simulink model "induction_machine_qd0"  (R2021b)
settings: Solver=FixedStepDiscrete  StartTime=0.0  StopTime=0.5  FixedStep=Ts  RelTol=1e-3
InitFcn:
  | Ts=1e-5;
  | Fe=50;
  | Vrms=230;
undefined symbols (not defined in the file): DiscIntNeverNeededParam
settings Model: Creator=lecci  LastModifiedBy=lecci

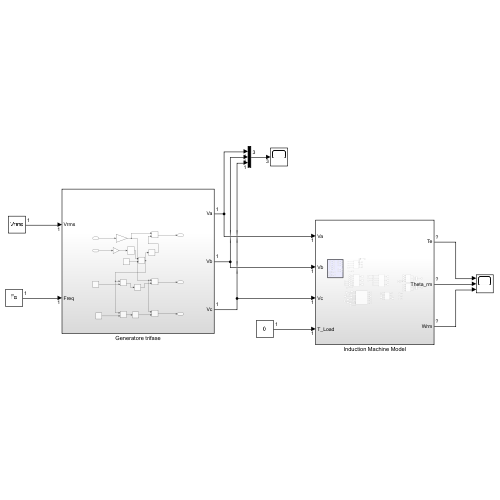
[thumbnail: Simulink's stored preview of the top-level diagram]
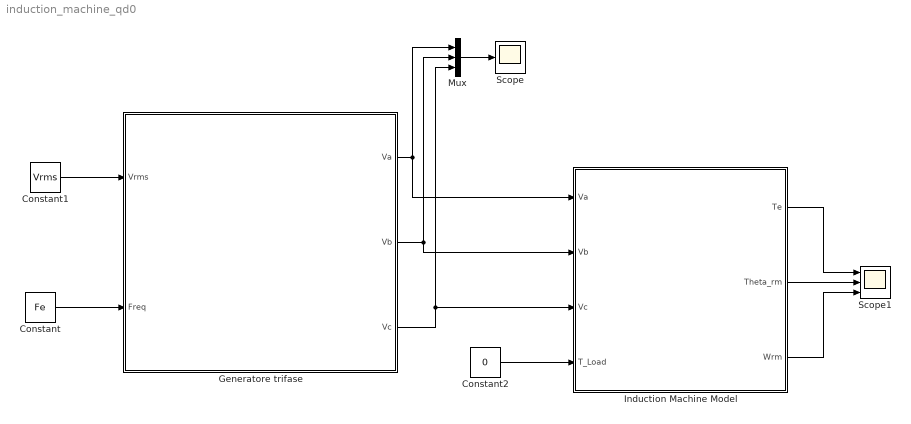
== system induction_machine_qd0 ==
  Constant : Constant  Value=Fe
  Constant1 : Constant  Value=Vrms
  Constant2 : Constant  Value=0
  Generatore trifase : Subsystem
  Induction Machine Model : Subsystem
  Mux : Mux  Inputs=3
  Scope : Scope
  Scope1 : Scope  NumInputPorts=3
  wires:
  Constant/1 -> Generatore trifase/2(Freq)
  Constant1/1 -> Generatore trifase/1(Vrms)
  Generatore trifase/1(Va) -> Induction Machine Model/1(Va), Mux/1
  Generatore trifase/2(Vb) -> Induction Machine Model/2(Vb), Mux/2
  Generatore trifase/3(Vc) -> Induction Machine Model/3(Vc), Mux/3
  Mux/1 -> Scope/1
  Constant2/1 -> Induction Machine Model/4(T_Load)
  Induction Machine Model/2(Theta_rm) -> Scope1/2
  Induction Machine Model/1(Te) -> Scope1/1
  Induction Machine Model/3(Wrm) -> Scope1/3

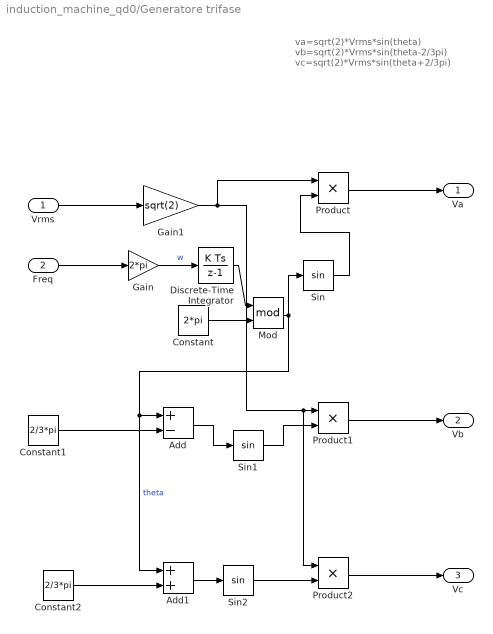
== system induction_machine_qd0/Generatore trifase ==
  note: va=sqrt(2)*Vrms*sin(theta)
      | vb=sqrt(2)*Vrms*sin(theta-2/3pi)
      | vc=sqrt(2)*Vrms*sin(theta+2/3pi)
  Vrms : Inport
  Freq : Inport  Port=2
  Add : Sum  Inputs=+-
  Add1 : Sum
  Constant : Constant  Value=2*pi
  Constant1 : Constant  Value=2/3*pi
  Constant2 : Constant  Value=2/3*pi
  Discrete-Time Integrator : DiscreteIntegrator  SampleTime=-1  ICPrevOutput=DiscIntNeverNeededParam  ICPrevScaledInput=DiscIntNeverNeededParam
  Gain : Gain  Gain=2*pi
  Gain1 : Gain  Gain=sqrt(2)
  Mod : Math  Operator=mod  SaturateOnIntegerOverflow=on
  Product : Product
  Product1 : Product
  Product2 : Product
  Sin : Trigonometry
  Sin1 : Trigonometry
  Sin2 : Trigonometry
  Va : Outport
  Vb : Outport  Port=2
  Vc : Outport  Port=3
  wires:
  Freq/1 -> Gain/1
  Constant/1 -> Mod/2
  Gain/1 -> Discrete-Time Integrator/1  "w"
  Discrete-Time Integrator/1 -> Mod/1
  Mod/1 -> Add1/1, Add/1, Sin/1  "theta"
  Sin/1 -> Product/2
  Product/1 -> Va/1
  Constant1/1 -> Add/2
  Product1/1 -> Vb/1
  Product2/1 -> Vc/1
  Constant2/1 -> Add1/2
  Gain1/1 -> Product2/1, Product1/1, Product/1
  Vrms/1 -> Gain1/1
  Add/1 -> Sin1/1
  Sin1/1 -> Product1/2
  Add1/1 -> Sin2/1
  Sin2/1 -> Product2/2

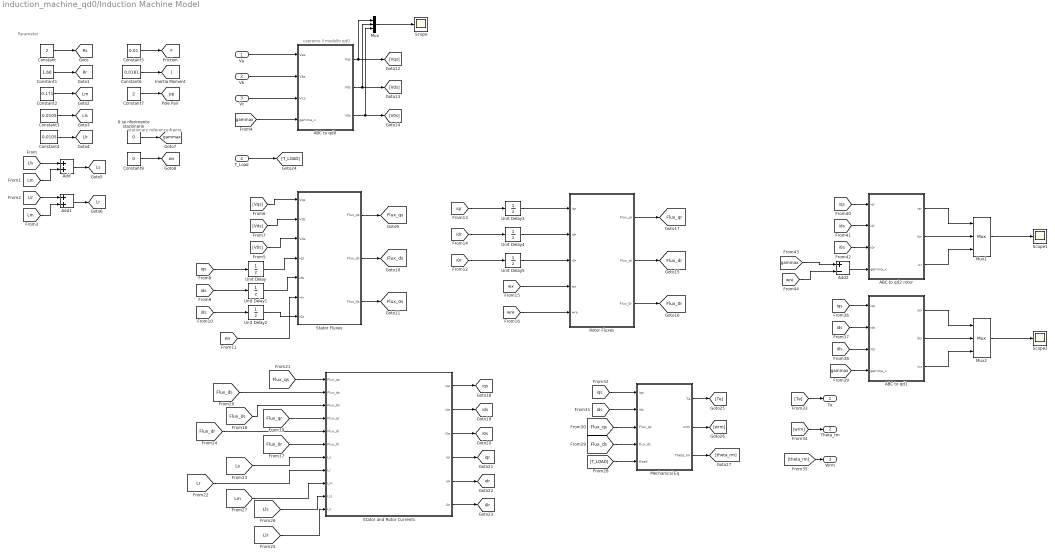
== system induction_machine_qd0/Induction Machine Model ==
  note: stationary reference frame
  note: useremo il modello qd0
  note: Parameter
  Va : Inport
  Vb : Inport  Port=2
  Vc : Inport  Port=3
  T_Load : Inport  Port=4
  0 se riferimento stazionario : Constant  Value=0
  ABC to qd0 : MATLAB Function  TreatAsAtomicUnit=on
  ABC to qd1 : MATLAB Function  TreatAsAtomicUnit=on
  ABC to qd2 rotor : MATLAB Function  TreatAsAtomicUnit=on
  Add : Sum
  Add1 : Sum
  Add2 : Sum  Inputs=+-
  Constant : Constant  Value=2
  Constant1 : Constant  Value=1.66
  Constant2 : Constant  Value=0.171
  Constant3 : Constant  Value=0.0105
  Constant4 : Constant  Value=0.0105
  Constant5 : Constant  Value=0.01
  Constant6 : Constant  Value=0.0181
  Constant7 : Constant  Value=2
  Constant9 : Constant  Value=0
  Mechanical Eq : Subsystem
  Mux : Mux  Inputs=3
  Mux1 : Mux  Inputs=3
  Mux2 : Mux  Inputs=3
  Rotor Fluxes : Subsystem
  Scope : Scope
  Scope1 : Scope
  Scope2 : Scope
  Stator Fluxes : Subsystem
  Stator and Rotor Currents : MATLAB Function  TreatAsAtomicUnit=on
  Unit Delay{,1..5} (6 alike) : UnitDelay  SampleTime=-1  HasFrameUpgradeWarning=on
  Te : Outport
  Theta_rm : Outport  Port=2
  Wrm : Outport  Port=3
  tag scope: F=global, Flux_0r=global, Flux_0s=global, Flux_dr=global, Flux_ds=global, Flux_qr=global, Flux_qs=global, J=global, Llr=global, Lls=global, Lm=global, Lr=global, Ls=global, Rr=global, Rs=global, gammax=global, i0r=global, i0s=global, idr=global, ids=global, iqr=global, iqs=global, pp=global, wx=global
  wires:
  Constant/1 -> [Rs]
  Constant1/1 -> [Rr]
  Constant2/1 -> [Lm]
  Constant3/1 -> [Lls]
  Constant4/1 -> [Llr]
  Add/1 -> [Ls]
  [Lls] -> Add/1
  [Lm] -> Add/2
  Add1/1 -> [Lr]
  [Llr] -> Add1/1
  [Lm] -> Add1/2
  Constant5/1 -> [F]
  Constant6/1 -> [J]
  Constant7/1 -> [pp]
  Va/1 -> ABC to qd0/1(Vas)
  Vb/1 -> ABC to qd0/2(Vbs)
  Vc/1 -> ABC to qd0/3(Vcs)
  0 se riferimento stazionario/1 -> [gammax]
  [gammax] -> ABC to qd0/4(gamma_x)
  Constant9/1 -> [wx]
  ABC to qd0/1(Vqs) -> [Vqs], Mux/1
  ABC to qd0/2(Vds) -> [Vds], Mux/2
  ABC to qd0/3(V0s) -> [V0s], Mux/3
  Mux/1 -> Scope/1
  Stator Fluxes/1(Flux_qs) -> [Flux_qs]
  Stator Fluxes/2(Flux_ds) -> [Flux_ds]
  Stator Fluxes/3(Flux_0s) -> [Flux_0s]
  [V0s] -> Stator Fluxes/3(V0s)
  [Vqs] -> Stator Fluxes/1(Vqs)
  [Vds] -> Stator Fluxes/2(Vds)
  [i0s] -> Unit Delay2/1
  Unit Delay2/1 -> Stator Fluxes/7(i0s)
  [ids] -> Unit Delay1/1
  [iqs] -> Unit Delay/1
  Unit Delay/1 -> Stator Fluxes/4(iqs)
  Unit Delay1/1 -> Stator Fluxes/5(ids)
  [wx] -> Stator Fluxes/6(wx)
  [idr] -> Unit Delay4/1
  [i0r] -> Unit Delay5/1
  [iqr] -> Unit Delay3/1
  Unit Delay3/1 -> Rotor Fluxes/1(iqr)
  Unit Delay4/1 -> Rotor Fluxes/2(idr)
  Unit Delay5/1 -> Rotor Fluxes/3(i0r)
  [wx] -> Rotor Fluxes/4(wx)
  [wre] -> Rotor Fluxes/5(wre)
  Rotor Fluxes/1(Flux_qr) -> [Flux_qr]
  Rotor Fluxes/2(Flux_dr) -> [Flux_dr]
  Rotor Fluxes/3(Flux_0r) -> [Flux_0r]
  Stator and Rotor Currents/1(iqs) -> [iqs]
  Stator and Rotor Currents/3(i0s) -> [i0s]
  Stator and Rotor Currents/2(ids) -> [ids]
  Stator and Rotor Currents/4(iqr) -> [iqr]
  Stator and Rotor Currents/5(idr) -> [idr]
  Stator and Rotor Currents/6(i0r) -> [i0r]
  [Flux_0r] -> Stator and Rotor Currents/6(Flux_0r)
  [Flux_ds] -> Stator and Rotor Currents/2(Flux_ds)
  [Flux_qs] -> Stator and Rotor Currents/1(Flux_qs)
  [Flux_0s] -> Stator and Rotor Currents/3(Flux_0s)
  [Flux_qr] -> Stator and Rotor Currents/4(Flux_qr)
  [Flux_dr] -> Stator and Rotor Currents/5(Flux_dr)
  [Ls] -> Stator and Rotor Currents/7(Ls)
  [Lr] -> Stator and Rotor Currents/8(Lr)
  [Lm] -> Stator and Rotor Currents/9(Lm)
  [Lls] -> Stator and Rotor Currents/10(Lls)
  [Llr] -> Stator and Rotor Currents/11(Llr)
  T_Load/1 -> [T_LOAD]
  [T_LOAD] -> Mechanical Eq/5(tload)
  [Flux_ds] -> Mechanical Eq/4(flux_ds)
  [Flux_qs] -> Mechanical Eq/3(Flux_qs)
  [ids] -> Mechanical Eq/2(ids)
  [iqs] -> Mechanical Eq/1(iqs)
  Mechanical Eq/1(Te) -> [Te]
  Mechanical Eq/2(wrm) -> [wrm]
  Mechanical Eq/3(Theta_rm) -> [theta_rm]
  [Te] -> Te/1
  [wrm] -> Theta_rm/1
  [theta_rm] -> Wrm/1
  [iqs] -> ABC to qd1/1(iqs)
  [ids] -> ABC to qd1/2(ids)
  [i0s] -> ABC to qd1/3(i0s)
  [gammax] -> ABC to qd1/4(gamma_x)
  [iqs] -> ABC to qd2 rotor/1(iqr)
  [ids] -> ABC to qd2 rotor/2(idr)
  [i0s] -> ABC to qd2 rotor/3(i0r)
  ABC to qd2 rotor/1(iar) -> Mux1/1
  ABC to qd2 rotor/2(ibr) -> Mux1/2
  ABC to qd2 rotor/3(icr) -> Mux1/3
  Mux1/1 -> Scope1/1
  ABC to qd1/3(ics) -> Mux2/3
  Mux2/1 -> Scope2/1
  ABC to qd1/2(ibs) -> Mux2/2
  ABC to qd1/1(ias) -> Mux2/1
  Add2/1 -> ABC to qd2 rotor/4(gamma_x)
  [gammax] -> Add2/1
  [wre] -> Add2/2

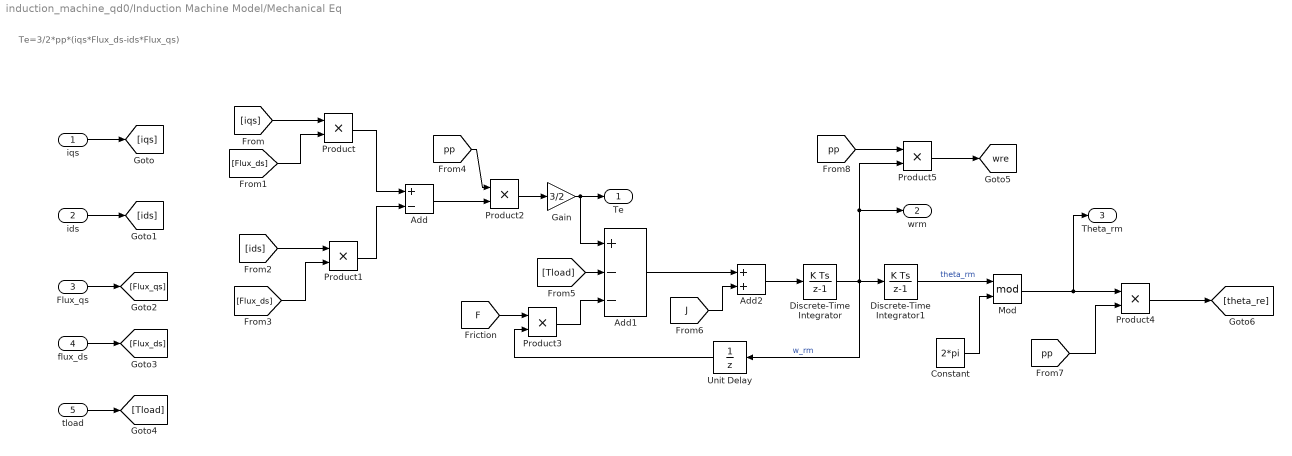
== system induction_machine_qd0/Induction Machine Model/Mechanical Eq ==
  note: Te=3/2*pp*(iqs*Flux_ds-ids*Flux_qs)
  iqs : Inport
  ids : Inport  Port=2
  Flux_qs : Inport  Port=3
  flux_ds : Inport  Port=4
  tload : Inport  Port=5
  Add : Sum  Inputs=+-
  Add1 : Sum  Inputs=+--
  Add2 : Sum
  Constant : Constant  Value=2*pi
  Discrete-Time Integrator : DiscreteIntegrator  SampleTime=-1  ICPrevOutput=DiscIntNeverNeededParam  ICPrevScaledInput=DiscIntNeverNeededParam
  Discrete-Time Integrator1 : DiscreteIntegrator  SampleTime=-1  ICPrevOutput=DiscIntNeverNeededParam  ICPrevScaledInput=DiscIntNeverNeededParam
  Gain : Gain  Gain=3/2
  Mod : Math  Operator=mod  SaturateOnIntegerOverflow=on
  Product{,1..5} (6 alike) : Product
  Unit Delay : UnitDelay  SampleTime=-1  HasFrameUpgradeWarning=on
  Te : Outport
  wrm : Outport  Port=2
  Theta_rm : Outport  Port=3
  tag scope: wre=global
  wires:
  iqs/1 -> [iqs]
  ids/1 -> [ids]
  Flux_qs/1 -> [Flux_qs]
  flux_ds/1 -> [Flux_ds]
  [iqs] -> Product/1
  [Flux_ds] -> Product/2
  Product/1 -> Add/1
  [Flux_ds] -> Product1/2
  [ids] -> Product1/1
  Product1/1 -> Add/2
  Add/1 -> Product2/2
  [pp] -> Product2/1
  Product2/1 -> Gain/1
  Gain/1 -> Add1/1, Te/1
  tload/1 -> [Tload]
  [Tload] -> Add1/2
  Product3/1 -> Add1/3
  [F] -> Product3/1
  Add1/1 -> Add2/1
  [J] -> Add2/2
  Add2/1 -> Discrete-Time Integrator/1
  Discrete-Time Integrator/1 -> Product5/2, wrm/1, Discrete-Time Integrator1/1, Unit Delay/1  "w_rm"
  Unit Delay/1 -> Product3/2
  Constant/1 -> Mod/2
  Mod/1 -> Theta_rm/1, Product4/1
  [pp] -> Product4/2
  Discrete-Time Integrator1/1 -> Mod/1  "theta_rm"
  [pp] -> Product5/1
  Product5/1 -> [wre]
  Product4/1 -> [theta_re]

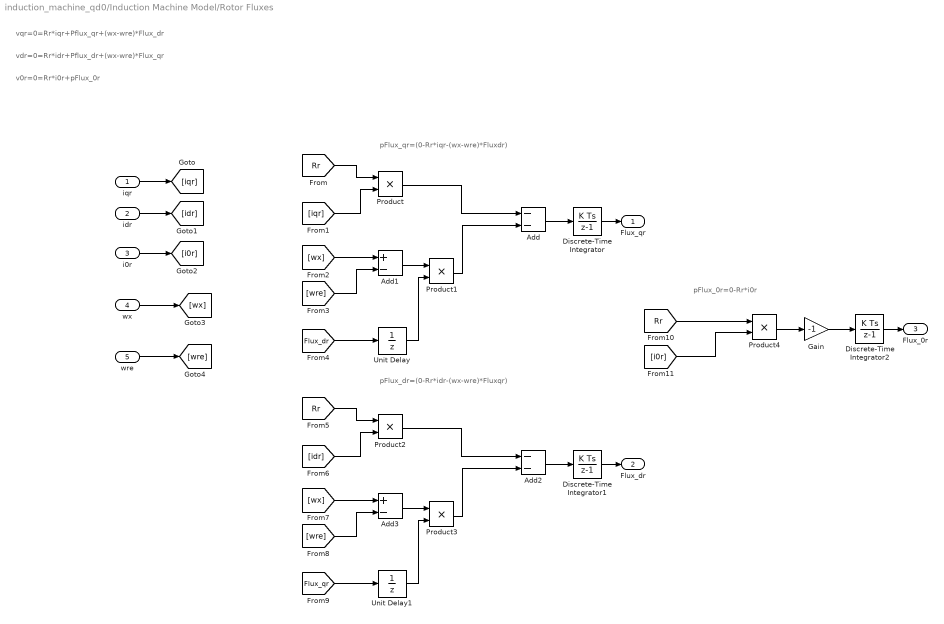
== system induction_machine_qd0/Induction Machine Model/Rotor Fluxes ==
  note: pFlux_0r=0-Rr*i0r
  note: pFlux_dr=(0-Rr*idr-(wx-wre)*Fluxqr)
  note: pFlux_qr=(0-Rr*iqr-(wx-wre)*Fluxdr)
  note: v0r=0=Rr*i0r+pFlux_0r
  note: vdr=0=Rr*idr+Pflux_dr+(wx-wre)*Flux_qr
  note: vqr=0=Rr*iqr+Pflux_qr+(wx-wre)*Flux_dr
  iqr : Inport
  idr : Inport  Port=2
  i0r : Inport  Port=3
  wx : Inport  Port=4
  wre : Inport  Port=5
  Add : Sum  Inputs=--
  Add1 : Sum  Inputs=+-
  Add2 : Sum  Inputs=--
  Add3 : Sum  Inputs=+-
  Discrete-Time Integrator : DiscreteIntegrator  SampleTime=-1  ICPrevOutput=DiscIntNeverNeededParam  ICPrevScaledInput=DiscIntNeverNeededParam
  Discrete-Time Integrator1 : DiscreteIntegrator  SampleTime=-1  ICPrevOutput=DiscIntNeverNeededParam  ICPrevScaledInput=DiscIntNeverNeededParam
  Discrete-Time Integrator2 : DiscreteIntegrator  SampleTime=-1  ICPrevOutput=DiscIntNeverNeededParam  ICPrevScaledInput=DiscIntNeverNeededParam
  Gain : Gain  Gain=-1
  Product{,1..4} (5 alike) : Product
  Unit Delay : UnitDelay  SampleTime=-1  HasFrameUpgradeWarning=on
  Unit Delay1 : UnitDelay  SampleTime=-1  HasFrameUpgradeWarning=on
  Flux_qr : Outport
  Flux_dr : Outport  Port=2
  Flux_0r : Outport  Port=3
  wires:
  iqr/1 -> [iqr]
  idr/1 -> [idr]
  i0r/1 -> [i0r]
  wx/1 -> [wx]
  wre/1 -> [wre]
  [Rr] -> Product/1
  [iqr] -> Product/2
  Product/1 -> Add/1
  [wx] -> Add1/1
  [wre] -> Add1/2
  Add1/1 -> Product1/1
  Product1/1 -> Add/2
  Add/1 -> Discrete-Time Integrator/1
  Discrete-Time Integrator/1 -> Flux_qr/1
  Product3/1 -> Add2/2
  Product2/1 -> Add2/1
  [wx] -> Add3/1
  Discrete-Time Integrator1/1 -> Flux_dr/1
  [wre] -> Add3/2
  [Rr] -> Product2/1
  Add2/1 -> Discrete-Time Integrator1/1
  [idr] -> Product2/2
  Add3/1 -> Product3/1
  Discrete-Time Integrator2/1 -> Flux_0r/1
  Gain/1 -> Discrete-Time Integrator2/1
  Product4/1 -> Gain/1
  [Rr] -> Product4/1
  [i0r] -> Product4/2
  Unit Delay/1 -> Product1/2
  [Flux_dr] -> Unit Delay/1
  [Flux_qr] -> Unit Delay1/1
  Unit Delay1/1 -> Product3/2

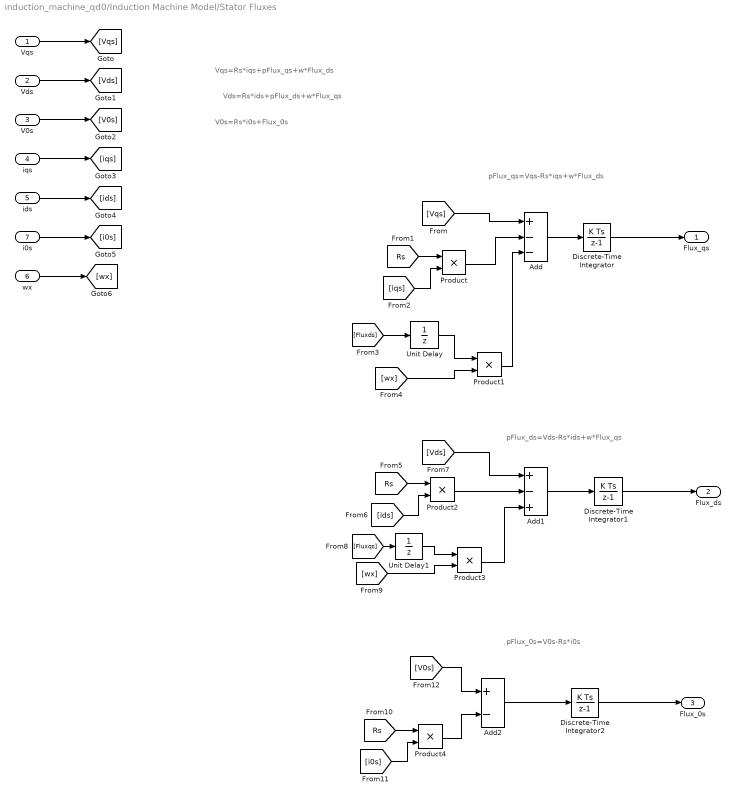
== system induction_machine_qd0/Induction Machine Model/Stator Fluxes ==
  note: pFlux_0s=V0s-Rs*i0s
  note: pFlux_qs=Vqs-Rs*iqs+w*Flux_ds
  note: pFlux_ds=Vds-Rs*ids+w*Flux_qs
  note: V0s=Rs*i0s+Flux_0s
  note: Vds=Rs*ids+pFlux_ds+w*Flux_qs
  note: Vqs=Rs*iqs+pFlux_qs+w*Flux_ds
  Vqs : Inport
  Vds : Inport  Port=2
  V0s : Inport  Port=3
  iqs : Inport  Port=4
  ids : Inport  Port=5
  wx : Inport  Port=6
  i0s : Inport  Port=7
  Add : Sum  Inputs=+--
  Add1 : Sum  Inputs=+-+
  Add2 : Sum  Inputs=+-
  Discrete-Time Integrator : DiscreteIntegrator  SampleTime=-1  ICPrevOutput=DiscIntNeverNeededParam  ICPrevScaledInput=DiscIntNeverNeededParam
  Discrete-Time Integrator1 : DiscreteIntegrator  SampleTime=-1  ICPrevOutput=DiscIntNeverNeededParam  ICPrevScaledInput=DiscIntNeverNeededParam
  Discrete-Time Integrator2 : DiscreteIntegrator  SampleTime=-1  ICPrevOutput=DiscIntNeverNeededParam  ICPrevScaledInput=DiscIntNeverNeededParam
  Product{,1..4} (5 alike) : Product
  Unit Delay : UnitDelay  SampleTime=-1  HasFrameUpgradeWarning=on
  Unit Delay1 : UnitDelay  SampleTime=-1  HasFrameUpgradeWarning=on
  Flux_qs : Outport
  Flux_ds : Outport  Port=2
  Flux_0s : Outport  Port=3
  wires:
  Vqs/1 -> [Vqs]
  V0s/1 -> [V0s]
  iqs/1 -> [iqs]
  ids/1 -> [ids]
  i0s/1 -> [i0s]
  [Vqs] -> Add/1
  [Rs] -> Product/1
  [iqs] -> Product/2
  Product/1 -> Add/2
  [wx] -> Product1/2
  [Fluxds] -> Unit Delay/1
  Unit Delay/1 -> Product1/1
  Product1/1 -> Add/3
  Add/1 -> Discrete-Time Integrator/1
  Discrete-Time Integrator/1 -> Flux_qs/1
  [Rs] -> Product2/1
  [ids] -> Product2/2
  Product2/1 -> Add1/2
  [Vds] -> Add1/1
  [Fluxqs] -> Unit Delay1/1
  [wx] -> Product3/2
  Unit Delay1/1 -> Product3/1
  Product3/1 -> Add1/3
  Discrete-Time Integrator1/1 -> Flux_ds/1
  Add1/1 -> Discrete-Time Integrator1/1
  Add2/1 -> Discrete-Time Integrator2/1
  Discrete-Time Integrator2/1 -> Flux_0s/1
  [i0s] -> Product4/2
  [Rs] -> Product4/1
  [V0s] -> Add2/1
  Product4/1 -> Add2/2
  Vds/1 -> [Vds]
  wx/1 -> [wx]

== matlab function induction_machine_qd0/Induction Machine Model/Stator and Rotor Currents ==
  data: Flux_qs input; iqs output; Flux_ds input; Flux_0s input; Flux_qr input; Flux_dr input; Flux_0r input; Ls input; Lr input; Lm input; ids output; i0s output; iqr output; idr output; i0r output; Lls input; Llr input
function [iqs,ids,i0s,iqr,idr,i0r] = fcn(Flux_qs,Flux_ds,Flux_0s,Flux_qr,Flux_dr,Flux_0r,Ls,Lr,Lm,Lls,Llr)

Flux=[Flux_qs; Flux_ds;Flux_qr;Flux_dr]

L=[Ls 0 Lm 0;
    0 Ls 0 Lm;
    Lm 0 Lr 0;
    0 Lm 0 Lr]

iqd=inv(L)*Flux;

iqs=idq(1);
ids=iqd(2);
iqr=iqd(3);
idr=iqd(4);

i0s=Flux_0s/Lls;
i0r=Flux_0r/Llr;

== matlab function induction_machine_qd0/Induction Machine Model/ABC to qd0 ==
  data: Vas input; Vqs output; Vbs input; Vcs input; gamma_x input; Vds output; V0s output
function [Vqs,Vds,V0s] = fcn(Vas,Vbs,Vcs,gamma_x)

Vabcs=[Vas;Vbs;Vcs];

K=2/3*[cos(gamma_x) cos(gamma_x-2/3*pi) cos(gamma_x+2/3*pi);
       sin(gamma_x) sin(gamma_x-2/3*pi) sin(gamma_x+2/3*pi);
       1/2                1/2                1/2     ];

Vqds=K*Vabcs;

Vqs=Vqds(1);
Vds=Vqds(2);
V0s=Vqds(3);

== matlab function induction_machine_qd0/Induction Machine Model/ABC to qd1 ==
  data: iqs input; ias output; ids input; i0s input; gamma_x input; ibs output; ics output
function [ias,ibs,ics] = fcn(iqs,ids,i0s,gamma_x)

Iqd0s=[iqs;ids;i0s];

invK=[cos(gamma_x) sin(gamma_x) 1;
       cos(gamma_x-2/3*pi) sin(gamma_x-2/3*pi) 1;
       cos(gamma_x+2/3*pi) sin(gamma_x+2/3*pi) 1];

Iabcs=invK*Iqd0s;

ias=Iabcs(1);
ibs=Iabcs(2);
ics=Iabcs(3);

== matlab function induction_machine_qd0/Induction Machine Model/ABC to qd2 rotor ==
  data: iqr input; iar output; idr input; i0r input; gamma_x input; ibr output; icr output
function [iar,ibr,icr] = fcn(iqr,idr,i0r,gamma_x)

Iqd0r=[iqr;idr;i0r];

invK=[cos(gamma_x) sin(gamma_x) 1;
       cos(gamma_x-2/3*pi) sin(gamma_x-2/3*pi) 1;
       cos(gamma_x+2/3*pi) sin(gamma_x+2/3*pi) 1];

Iabcr=invK*Iqd0r;

iar=Iabcr(1);
ibr=Iabcr(2);
icr=Iabcr(3);
